simulink model "controller_loop"  (Simulink 8.1)
settings: Solver=ode45  StartTime=0.0  StopTime=10.0  RelTol=1e-3
values from neighbouring files (symbols this model uses):
  A = [1.5 0.5;0.5 1.0]    [controller_s.m]    (also in controller_us.m)
  B = [2; 0]    [controller_s.m]    (also in controller_us.m)
  K = place(A,B,des_con)    [controller_s.m]    (also in controller_us.m = -K)
  P = dlyap((A-B*K)',Q)    [controller_s.m]    (also in controller_us.m)
settings Model: Creator=dejanira  LastModifiedBy=dejanira
settings DataIOCC: SignalLoggingSaveFormat=Dataset
settings OptimizationCC: ExpressionDepthLimit=128
settings DebuggingCC: FcnCallInpInsideContextMsg=EnableAllAsError
settings GRTTargetCC: CombineOutputUpdateFcns=on  GRTInterface=off

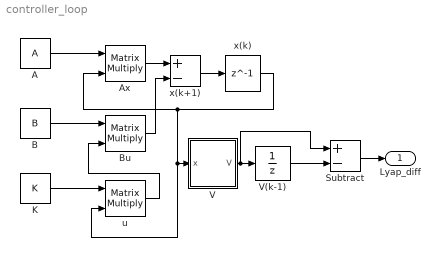
== system controller_loop ==
  A : Constant  Value=A  VectorParams1D=off
  Ax : Product  Multiplication=Matrix(*)  SampleTime=0.1
  B : Constant  Value=B  VectorParams1D=off
  Bu : Product  Multiplication=Matrix(*)  SampleTime=0.1
  K : Constant  Value=K  VectorParams1D=off
  Subtract : Sum  Inputs=+-
  V : Subsystem
      mask Display: disp('x^TPx')
  V(k-1) : UnitDelay  InitialCondition=100000  SampleTime=0.01
  u : Product  Multiplication=Matrix(*)  SampleTime=0.1
  x(k) : Delay  DelayLength=1  InitialCondition=1
  x(k+1) : Sum  Inputs=+-
  Lyap_diff : Outport
  wires:
  x(k)/1 -> u/2, V/1(x), Ax/2
  B/1 -> Bu/1
  Ax/1 -> x(k+1)/1
  K/1 -> u/1
  Bu/1 -> x(k+1)/2
  A/1 -> Ax/1
  u/1 -> Bu/2
  V/1(V) -> Subtract/1, V(k-1)/1
  x(k+1)/1 -> x(k)/1
  V(k-1)/1 -> Subtract/2
  Subtract/1 -> Lyap_diff/1

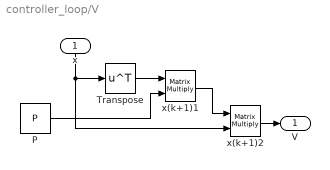
== system controller_loop/V ==
  x : Inport
  P : Constant  Value=P
  Transpose : Math  Operator=transpose  SaturateOnIntegerOverflow=on
  x(k+1)1 : Product  Multiplication=Matrix(*)
  x(k+1)2 : Product  Multiplication=Matrix(*)
  V : Outport
  wires:
  Transpose/1 -> x(k+1)1/1
  x(k+1)1/1 -> x(k+1)2/1
  x/1 -> x(k+1)2/2, Transpose/1
  x(k+1)2/1 -> V/1
  P/1 -> x(k+1)1/2
